simulink model "LQR_test"  (R2017b)
settings: Solver=ode4  StartTime=0.0  StopTime=10  FixedStep=1e-3  RelTol=1e-3  EnableMultiTasking=on
values from neighbouring files (symbols this model uses):
  par =     [sim.mat]
libraries: Delft_Tyre_dtlib x1, Delft_Tyre_sm1glib x1, simulink x1
settings Model: Creator=bshyrokau  LastModifiedBy=varun
settings DataIOCC: SaveOutput=off  SignalLogging=off  DSMLogging=off  SaveTime=off
settings OptimizationCC: LifeSpan=inf
settings DebuggingCC: AllowSymbolicDim=off  SFUnexpectedBacktrackingDiag=warning  SFNoUnconditionalDefaultTransitionDiag=warning  SFExecutionAtInitializationDiag=none
settings ModelReferenceCC: PropagateSignalLabelsOutOfModel=off
settings CodeAppCC: StateflowObjectComments=on
settings GRTTargetCC: TargetLangStandard=C89/C90 (ANSI)
settings ConfigComp: CovMetricSettings=dw  CovHtmlReporting=on  CovSaveCumulativeToWorkspaceVar=on  CovSaveSingleToWorkspaceVar=on  CovExternalEMLEnable=off

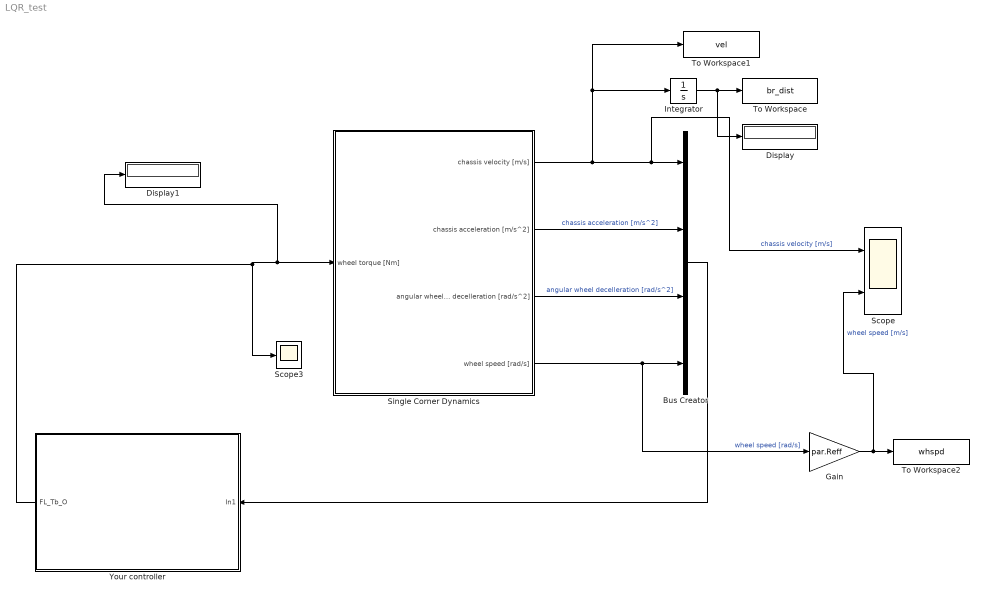
== system LQR_test ==
  Bus Creator : BusCreator  Inputs=4
  Display : Display
  Display1 : Display
  Gain : Gain  Gain=par.Reff
  Integrator : Integrator
  Scope : Scope  NumInputPorts=2
  Scope3 : Scope
  Single Corner Dynamics : Subsystem
  To Workspace : ToWorkspace  VariableName=br_dist  SaveFormat=Timeseries  SampleTime=-1
  To Workspace1 : ToWorkspace  VariableName=vel  SaveFormat=Timeseries  SampleTime=-1
  To Workspace2 : ToWorkspace  VariableName=whspd  SaveFormat=Timeseries  SampleTime=-1
  Your controller : Subsystem
  wires:
  Your controller/1(FL_Tb_O) -> Display1/1, Single Corner Dynamics/1(wheel torque [Nm]), Scope3/1
  Single Corner Dynamics/1(chassis velocity [m/s]) -> Scope/1, Bus Creator/1, To Workspace1/1, Integrator/1  "chassis velocity [m/s]"
  Single Corner Dynamics/2(chassis acceleration [m/s^2]) -> Bus Creator/2  "chassis acceleration [m/s^2]"
  Single Corner Dynamics/3(angular wheel decelleration [rad/s^2]) -> Bus Creator/3  "angular wheel decelleration [rad/s^2]"
  Single Corner Dynamics/4(wheel speed [rad/s]) -> Gain/1, Bus Creator/4  "wheel speed [rad/s]"
  Bus Creator/1 -> Your controller/1(In1)
  Integrator/1 -> Display/1, To Workspace/1
  Gain/1 -> Scope/2, To Workspace2/1  "wheel speed [m/s]"

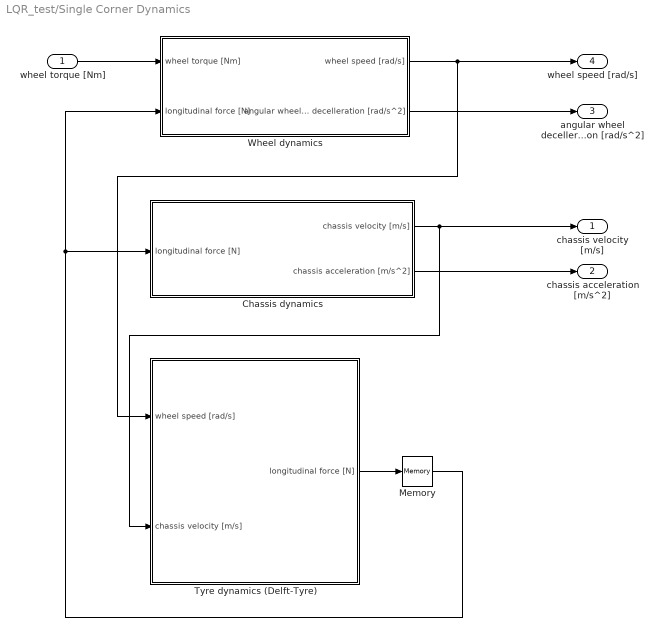
== system LQR_test/Single Corner Dynamics ==
  wheel torque [Nm] : Inport
  Chassis dynamics : Subsystem
  Memory : Memory
  Tyre dynamics (Delft-Tyre) : Subsystem
  Wheel dynamics : Subsystem
  chassis velocity [m/s] : Outport  VectorParamsAs1DForOutWhenUnconnected=off
  chassis acceleration [m/s^2] : Outport  Port=2  VectorParamsAs1DForOutWhenUnconnected=off
  angular wheel decelleration [rad/s^2] : Outport  Port=3  VectorParamsAs1DForOutWhenUnconnected=off
  wheel speed [rad/s] : Outport  Port=4  VectorParamsAs1DForOutWhenUnconnected=off
  wires:
  wheel torque [Nm]/1 -> Wheel dynamics/1(wheel torque [Nm])
  Wheel dynamics/1(wheel speed [rad/s]) -> Tyre dynamics (Delft-Tyre)/1(wheel speed [rad/s]), wheel speed [rad/s]/1
  Chassis dynamics/1(chassis velocity [m/s]) -> Tyre dynamics (Delft-Tyre)/2(chassis velocity [m/s]), chassis velocity [m/s]/1
  Tyre dynamics (Delft-Tyre)/1(longitudinal force [N]) -> Memory/1
  Memory/1 -> Wheel dynamics/2(longitudinal force [N]), Chassis dynamics/1(longitudinal force [N])
  Wheel dynamics/2(angular wheel decelleration [rad/s^2]) -> angular wheel decelleration [rad/s^2]/1
  Chassis dynamics/2(chassis acceleration [m/s^2]) -> chassis acceleration [m/s^2]/1

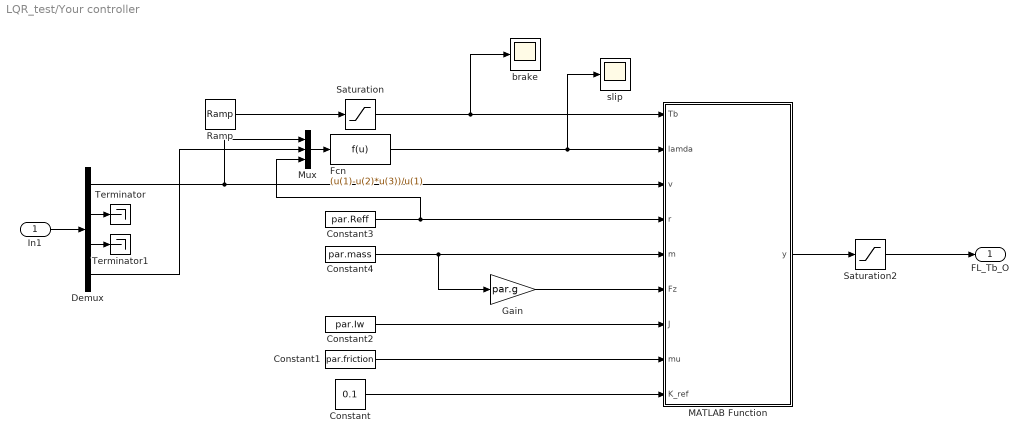
== system LQR_test/Your controller ==
  In1 : Inport
  Constant : Constant  Value=0.1
  Constant1 : Constant  Value=par.friction
  Constant2 : Constant  Value=par.Iw
  Constant3 : Constant  Value=par.Reff
  Constant4 : Constant  Value=par.mass
  Demux : Demux
  Fcn : Fcn  Expr=(u(1)-u(2)*u(3))/u(1)
  Gain : Gain  Gain=par.g
  MATLAB Function : MATLAB Function  TreatAsAtomicUnit=on
  Mux : Mux  Inputs=3
  Ramp : simulink/Sources/Ramp  slope=1136  start=2  X0=0
  Saturation : Saturate  UpperLimit=1136  LowerLimit=0
  Saturation2 : Saturate  UpperLimit=1136  LowerLimit=0
  Terminator : Terminator
  Terminator1 : Terminator
  brake : Scope
  slip : Scope
  FL_Tb_O : Outport  VectorParamsAs1DForOutWhenUnconnected=off
  wires:
  Constant4/1 -> Gain/1, MATLAB Function/5(m)
  Constant/1 -> MATLAB Function/9(K_ref)
  Constant3/1 -> Mux/3, MATLAB Function/4(r)
  Constant2/1 -> MATLAB Function/7(J)
  MATLAB Function/1(y) -> Saturation2/1
  Demux/1 -> Mux/1, MATLAB Function/3(v)
  Gain/1 -> MATLAB Function/6(Fz)
  Fcn/1 -> slip/1, MATLAB Function/2(lamda)
  Saturation/1 -> brake/1, MATLAB Function/1(Tb)
  Ramp/1 -> Saturation/1
  Constant1/1 -> MATLAB Function/8(mu)
  Demux/2 -> Terminator/1
  Demux/3 -> Terminator1/1
  In1/1 -> Demux/1
  Mux/1 -> Fcn/1
  Demux/4 -> Mux/2
  Saturation2/1 -> FL_Tb_O/1

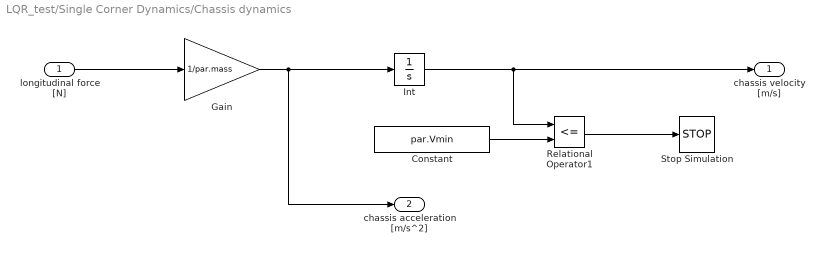
== system LQR_test/Single Corner Dynamics/Chassis dynamics ==
  longitudinal force [N] : Inport
  Constant : Constant  Value=par.Vmin
  Gain : Gain  Gain=1/par.mass
  Int : Integrator  InitialCondition=par.V0  LimitOutput=on  UpperSaturationLimit=200/3.6  LowerSaturationLimit=eps
  Relational Operator1 : RelationalOperator  Operator=<=  RndMeth=Nearest  InputSameDT=on
  Stop Simulation : Stop
  chassis velocity [m/s] : Outport  VectorParamsAs1DForOutWhenUnconnected=off
  chassis acceleration [m/s^2] : Outport  Port=2  VectorParamsAs1DForOutWhenUnconnected=off
  wires:
  longitudinal force [N]/1 -> Gain/1
  Int/1 -> Relational Operator1/1, chassis velocity [m/s]/1
  Gain/1 -> chassis acceleration [m/s^2]/1, Int/1
  Relational Operator1/1 -> Stop Simulation/1
  Constant/1 -> Relational Operator1/2

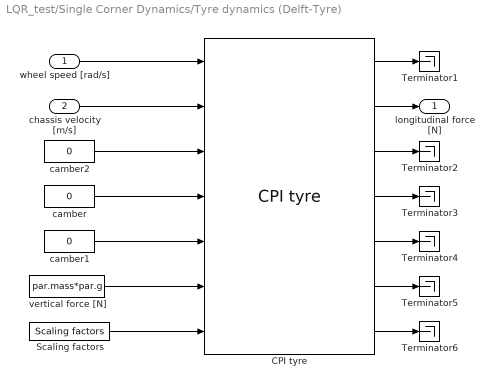
== system LQR_test/Single Corner Dynamics/Tyre dynamics (Delft-Tyre) ==
  wheel speed [rad/s] : Inport
  chassis velocity [m/s] : Inport  Port=2
  CPI tyre : Delft_Tyre_dtlib/Simulink/CPI tyre  Tag=CPI tyre  idtyre=1  tpfname='TNO_car205_60R15.tir'  side_mode=(3xxx) symmetric  dyn_mode=(xx1x) relaxation behaviour  mf_mode=(xxx1) longitudinal  use_mode=1e8  disp_debug=off
  Scaling factors : Delft_Tyre_sm1glib/SimMechanics 1G/Scaling factors  Tag=Scaling factors  LMUX=par.friction  LKX=1  LMUY=1  LKY=1  LKYC=1  LTR=1  LKZC=1
  Terminator{1..6} (6 alike) : Terminator
  camber : Constant  Value=0
  camber1 : Constant  Value=0
  camber2 : Constant  Value=0
  vertical force [N] : Constant  Value=par.mass*par.g
  longitudinal force [N] : Outport  VectorParamsAs1DForOutWhenUnconnected=off
  wires:
  Scaling factors/1 -> CPI tyre/7
  camber2/1 -> CPI tyre/3
  camber/1 -> CPI tyre/4
  CPI tyre/1 -> Terminator1/1
  CPI tyre/3 -> Terminator2/1
  CPI tyre/4 -> Terminator3/1
  CPI tyre/6 -> Terminator5/1
  CPI tyre/5 -> Terminator4/1
  camber1/1 -> CPI tyre/5
  chassis velocity [m/s]/1 -> CPI tyre/2
  wheel speed [rad/s]/1 -> CPI tyre/1
  CPI tyre/2 -> longitudinal force [N]/1
  vertical force [N]/1 -> CPI tyre/6
  CPI tyre/7 -> Terminator6/1

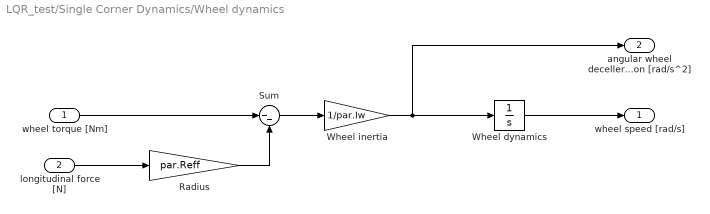
== system LQR_test/Single Corner Dynamics/Wheel dynamics ==
  wheel torque [Nm] : Inport
  longitudinal force [N] : Inport  Port=2
  Radius : Gain  Gain=par.Reff  SaturateOnIntegerOverflow=on  OutDataTypeStr=Inherit: Same as input  ParamDataTypeStr=Inherit: Same as input
  Sum : Sum  Inputs=|--  SaturateOnIntegerOverflow=on  InputSameDT=on  OutDataTypeStr=Inherit: Same as first input
  Wheel dynamics : Integrator  InitialCondition=par.V0/par.Reff  LimitOutput=on  UpperSaturationLimit=200/3.6/par.Reff  LowerSaturationLimit=eps
  Wheel inertia : Gain  Gain=1/par.Iw  SaturateOnIntegerOverflow=on  OutDataTypeStr=Inherit: Same as input  ParamDataTypeStr=Inherit: Same as input
  wheel speed [rad/s] : Outport  VectorParamsAs1DForOutWhenUnconnected=off
  angular wheel decelleration [rad/s^2] : Outport  Port=2  VectorParamsAs1DForOutWhenUnconnected=off
  wires:
  Wheel inertia/1 -> angular wheel decelleration [rad/s^2]/1, Wheel dynamics/1
  wheel torque [Nm]/1 -> Sum/1
  Wheel dynamics/1 -> wheel speed [rad/s]/1
  Sum/1 -> Wheel inertia/1
  longitudinal force [N]/1 -> Radius/1
  Radius/1 -> Sum/2

== matlab function LQR_test/Your controller/MATLAB Function ==
  data: Tb input; y output; lamda input; v input; r input; m input; Fz input; J input; mu input; K_ref input
function y = fcn(Tb, lamda, v, r, m, Fz, J, mu, K_ref)

alpha = ((1/m)*(1-K_ref)+(r^2/J))*Fz*mu;
beta = (r/J);
coder.extrinsic('lqr');
u = Tb;
if Tb > 0
    if v <= 1 
       K = [1,1];
    else
        A = [0 1;0 alpha/v];
        B = [0; beta/v];
        Q = 10000000*eye(2);
        R = 0.001;
        K = zeros(1,2);
        [K,~,~] = lqr(A,B,Q,R);
    end
    u = -K(2)*(lamda-K_ref);
end
y = u;
